simulink model "OdeModelling_SimplePendulumn"  (R2024a)
settings: Solver=VariableStepAuto  StartTime=0.0  StopTime=10.0  RelTol=1e-3
settings Model: Creator=JOJO  LastModifiedBy=JOJO

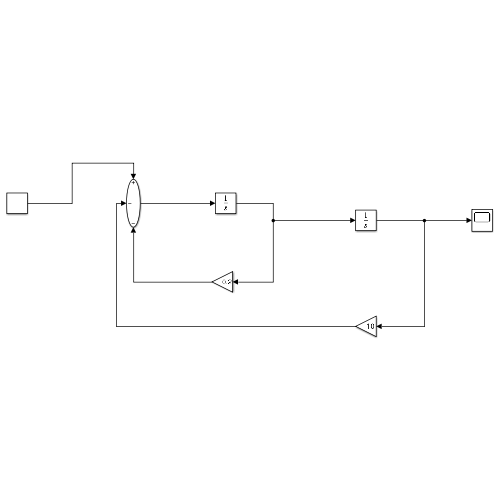
[thumbnail: Simulink's stored preview of the top-level diagram]
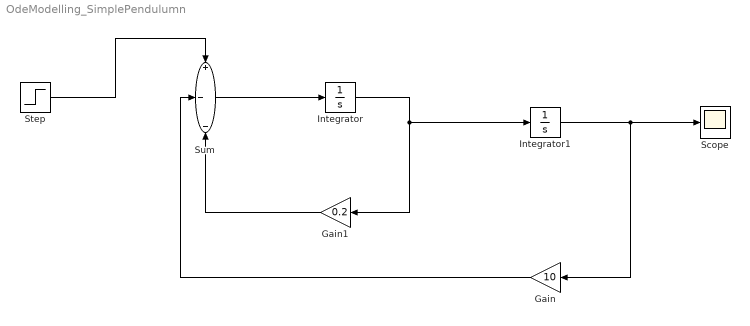
== system OdeModelling_SimplePendulumn ==
  Gain : Gain  Gain=10
  Gain1 : Gain  Gain=0.2
  Integrator : Integrator
  Integrator1 : Integrator
  Scope : Scope
  Step : Step  Time=3  SampleTime=0
  Sum : Sum  Inputs=+--
  wires:
  Integrator/1 -> Gain1/1, Integrator1/1
  Sum/1 -> Integrator/1
  Gain1/1 -> Sum/3
  Gain/1 -> Sum/2
  Integrator1/1 -> Gain/1, Scope/1
  Step/1 -> Sum/1
